simulink model "ex3_sim2"  (R2018b)
settings: Solver=ode45  StartTime=0.0  StopTime=0.5  MaxStep=0.001  RelTol=1e-3  EnableMultiTasking=on
undefined symbols (not defined in the file): Ar, degs2rpm, denC2d, denHd, DiscIntNeverNeededParam, k1, kawu, km, numC2d, numHd, rpm2rads, t0r, Tm, Ts
settings Model: Creator=antonello  LastModifiedBy=riccardo
settings DataIOCC: LimitDataPoints=on  SaveFormat=Array
settings OptimizationCC: LifeSpan=inf
settings DebuggingCC: SolverPrmCheckMsg=warning  LibraryContextMissingDiagnostic=none  SFUnexpectedBacktrackingDiag=warning  SFNoUnconditionalDefaultTransitionDiag=warning  SFExecutionAtInitializationDiag=none
settings HardwareCC: ProdBitPerPointer=32  ProdBitPerSizeT=32  ProdBitPerPtrDiffT=32  ProdLargestAtomicFloat=None  ProdIntDivRoundTo=Undefined  ProdEndianess=Unspecified  ProdWordSize=32  ProdHWDeviceType=32-bit Generic
settings ModelReferenceCC: PropagateSignalLabelsOutOfModel=off
settings SFSimCC: SimUseLocalCustomCode=off
settings RTWCC: RTWUseLocalCustomCode=off
settings CodeAppCC: StateflowObjectComments=on
settings GRTTargetCC: TargetLangStandard=C89/C90 (ANSI)  GeneratePreprocessorConditionals=Disable all
settings ConfigComp: CovMetricSettings=dw  CovHtmlReporting=on  CovSaveCumulativeToWorkspaceVar=on  CovSaveSingleToWorkspaceVar=on  CovExternalEMLEnable=off  CovSFcnEnable=off

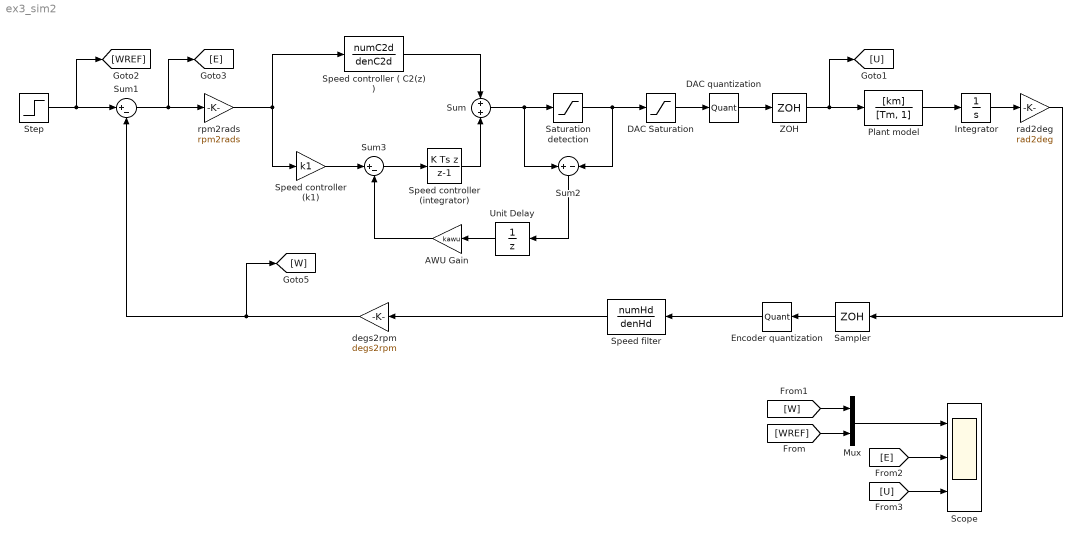
== system ex3_sim2 ==
  AWU Gain : Gain  Gain=kawu
  DAC Saturation : Saturate  UpperLimit=10  LowerLimit=-10
  DAC quantization : Quantizer  QuantizationInterval=qdac
  Encoder quantization : Quantizer  QuantizationInterval=qenc
  Integrator : Integrator
  Mux : Mux  Inputs=2
  Plant model : TransferFcn  Numerator=[km]  Denominator=[Tm, 1]
  Sampler : ZeroOrderHold  SampleTime=Ts
  Saturation detection : Saturate  UpperLimit=10  LowerLimit=-10
  Scope : Scope  NumInputPorts=3
  Speed controller (integrator) : DiscreteIntegrator  IntegratorMethod=Integration: Backward Euler  SampleTime=-1  ICPrevOutput=DiscIntNeverNeededParam  ICPrevScaledInput=DiscIntNeverNeededParam
  Speed controller ( C2(z) ) : DiscreteTransferFcn  Numerator=numC2d  Denominator=denC2d  SampleTime=Ts
  Speed controller (k1) : Gain  Gain=k1
  Speed filter : DiscreteTransferFcn  Numerator=numHd  Denominator=denHd
  Step : Step  Time=t0r  After=Ar  SampleTime=0
  Sum : Sum
  Sum1 : Sum  Inputs=|+-
  Sum2 : Sum  Inputs=+-
  Sum3 : Sum  Inputs=|+-
  Unit Delay : UnitDelay  SampleTime=-1
  ZOH : ZeroOrderHold  SampleTime=Ts
  degs2rpm : Gain  Gain=degs2rpm
  rad2deg : Gain  Gain=rad2deg
  rpm2rads : Gain  Gain=rpm2rads
  wires:
  Sum1/1 -> [E], rpm2rads/1
  Step/1 -> [WREF], Sum1/1
  [W] -> Mux/1
  [WREF] -> Mux/2
  DAC Saturation/1 -> DAC quantization/1
  Mux/1 -> Scope/1
  [E] -> Scope/2
  [U] -> Scope/3
  ZOH/1 -> Plant model/1, [U]
  Speed filter/1 -> degs2rpm/1
  degs2rpm/1 -> Sum1/2, [W]
  Plant model/1 -> Integrator/1
  Integrator/1 -> rad2deg/1
  rad2deg/1 -> Sampler/1
  DAC quantization/1 -> ZOH/1
  Sampler/1 -> Encoder quantization/1
  Encoder quantization/1 -> Speed filter/1
  Saturation detection/1 -> Sum2/2, DAC Saturation/1
  Sum/1 -> Sum2/1, Saturation detection/1
  Speed controller (integrator)/1 -> Sum/2
  Sum3/1 -> Speed controller (integrator)/1
  Speed controller ( C2(z) )/1 -> Sum/1
  rpm2rads/1 -> Speed controller (k1)/1, Speed controller ( C2(z) )/1
  Speed controller (k1)/1 -> Sum3/1
  Sum2/1 -> Unit Delay/1
  AWU Gain/1 -> Sum3/2
  Unit Delay/1 -> AWU Gain/1
